simulink model "pack_96s"  (R2024b)
settings: Solver=ode4  StartTime=0.0  StopTime=T_stop  FixedStep=0.1  RelTol=1e-3
undefined symbols (not defined in the file): cell_dSoC_pct, cell_Q_Ah, cell_RO_scale, cp_coolant, h_rad, m_coolant, P_chiller_max, P_heater_max, T_cells_init, tau_chiller, tau_heater
settings Model: Creator=rayen  LastModifiedBy=rayen
settings OptimizationCC: ZeroExternalMemoryAtStartup=off  ZeroInternalMemoryAtStartup=off
settings DebuggingCC: AlgebraicLoopMsg=error
settings SFSimCC: SimTargetLang=C++
settings RTWCC: TargetLang=C++
settings GRTTargetCC: TargetLangStandard=C++11 (ISO)  CodeInterfacePackaging=C++ class

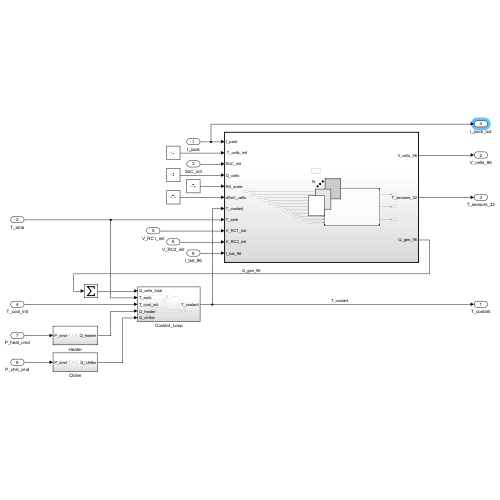
[thumbnail: Simulink's stored preview of the top-level diagram]
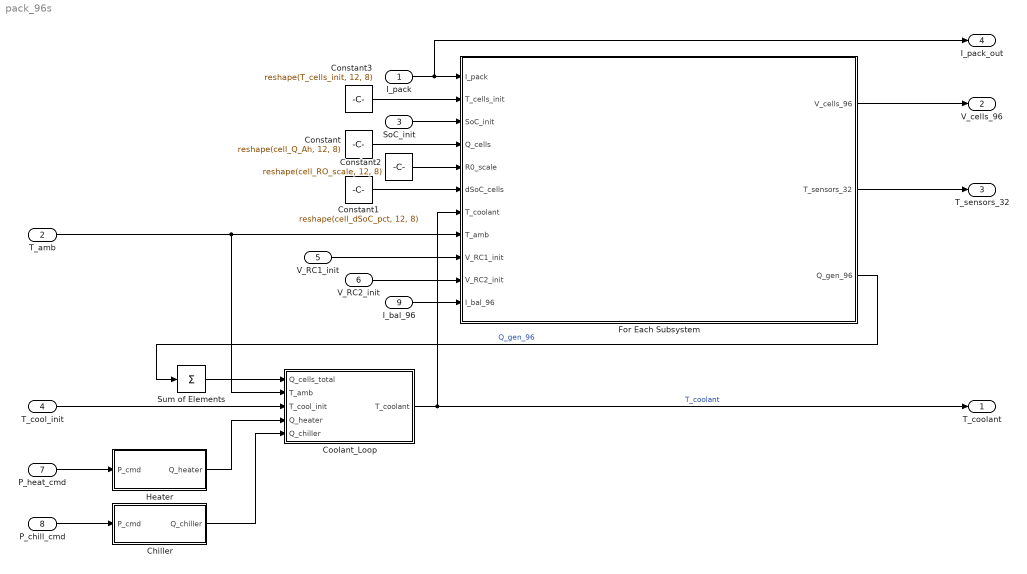
== system pack_96s ==
  I_pack : Inport  OutDataTypeStr=double
  T_amb : Inport  Port=2  OutDataTypeStr=double
  SoC_init : Inport  Port=3  OutDataTypeStr=double
  T_cool_init : Inport  Port=4  OutDataTypeStr=double
  V_RC1_init : Inport  Port=5  OutDataTypeStr=double
  V_RC2_init : Inport  Port=6  OutDataTypeStr=double
  P_heat_cmd : Inport  Port=7  OutDataTypeStr=double
  P_chill_cmd : Inport  Port=8  OutDataTypeStr=double
  I_bal_96 : Inport  Port=9  OutDataTypeStr=double
  Chiller : Subsystem
  Constant : Constant  Value=reshape(cell_Q_Ah, 12, 8)
  Constant1 : Constant  Value=reshape(cell_dSoC_pct, 12, 8)
  Constant2 : Constant  Value=reshape(cell_RO_scale, 12, 8)
  Constant3 : Constant  Value=reshape(T_cells_init, 12, 8)
  Coolant_Loop : Subsystem
  For Each Subsystem : Subsystem  TreatAsAtomicUnit=on
  Heater : Subsystem
  Sum of Elements : Sum  Inputs=+
  T_coolant : Outport  OutDataTypeStr=double
  V_cells_96 : Outport  Port=2  OutDataTypeStr=double
  T_sensors_32 : Outport  Port=3  OutDataTypeStr=double
  I_pack_out : Outport  Port=4  OutDataTypeStr=double
  wires:
  I_pack/1 -> I_pack_out/1, For Each Subsystem/1(I_pack)
  SoC_init/1 -> For Each Subsystem/3(SoC_init)
  Constant/1 -> For Each Subsystem/4(Q_cells)
  Constant2/1 -> For Each Subsystem/5(R0_scale)
  Constant1/1 -> For Each Subsystem/6(dSoC_cells)
  Sum of Elements/1 -> Coolant_Loop/1(Q_cells_total)
  Coolant_Loop/1(T_coolant) -> T_coolant/1, For Each Subsystem/7(T_coolant)  "T_coolant"
  Heater/1(Q_heater) -> Coolant_Loop/4(Q_heater)
  Chiller/1(Q_chiller) -> Coolant_Loop/5(Q_chiller)
  T_amb/1 -> For Each Subsystem/8(T_amb), Coolant_Loop/2(T_amb)
  T_cool_init/1 -> Coolant_Loop/3(T_cool_init)
  Constant3/1 -> For Each Subsystem/2(" T_cells_init")
  V_RC1_init/1 -> For Each Subsystem/9(V_RC1_init)
  V_RC2_init/1 -> For Each Subsystem/10(V_RC2_init)
  P_heat_cmd/1 -> Heater/1(P_cmd)
  P_chill_cmd/1 -> Chiller/1(P_cmd)
  For Each Subsystem/2(T_sensors_32) -> T_sensors_32/1
  For Each Subsystem/1(V_cells_96) -> V_cells_96/1
  For Each Subsystem/3(Q_gen_96) -> Sum of Elements/1  "Q_gen_96"
  I_bal_96/1 -> For Each Subsystem/11(I_bal_96)

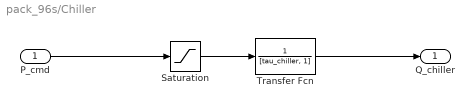
== system pack_96s/Chiller ==
  P_cmd : Inport
  Saturation : Saturate  UpperLimit=P_chiller_max  LowerLimit=0
  Transfer Fcn : TransferFcn  Denominator=[tau_chiller, 1]
  Q_chiller : Outport
  wires:
  Transfer Fcn/1 -> Q_chiller/1
  Saturation/1 -> Transfer Fcn/1
  P_cmd/1 -> Saturation/1

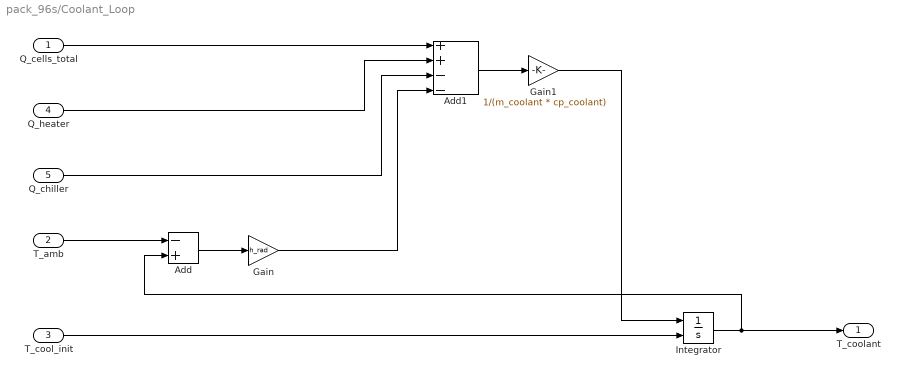
== system pack_96s/Coolant_Loop ==
  Q_cells_total : Inport
  T_amb : Inport  Port=2
  T_cool_init : Inport  Port=3
  Q_heater : Inport  Port=4
  Q_chiller : Inport  Port=5
  Add : Sum  Inputs=-+
  Add1 : Sum  Inputs=++--
  Gain : Gain  Gain=h_rad
  Gain1 : Gain  Gain=1/(m_coolant * cp_coolant)
  Integrator : Integrator  InitialConditionSource=external  LimitOutput=on  UpperSaturationLimit=80  LowerSaturationLimit=-40
  T_coolant : Outport
  wires:
  T_cool_init/1 -> Integrator/2
  Integrator/1 -> Add/2, T_coolant/1
  T_amb/1 -> Add/1
  Add/1 -> Gain/1
  Q_cells_total/1 -> Add1/1
  Q_heater/1 -> Add1/2
  Q_chiller/1 -> Add1/3
  Gain/1 -> Add1/4
  Add1/1 -> Gain1/1
  Gain1/1 -> Integrator/1

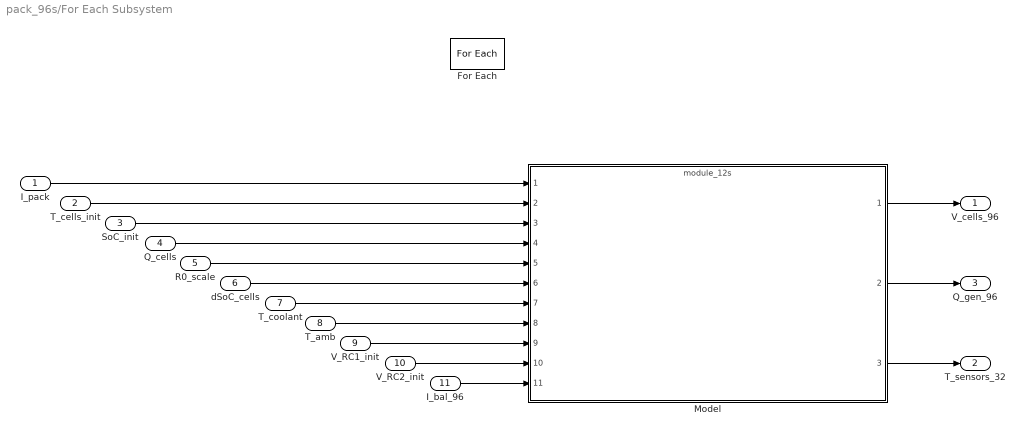
== system pack_96s/For Each Subsystem ==
  I_pack : Inport
  " T_cells_init" : Inport  Port=2  Partition=on  PartitionDimension=2  PartitionWidth=1  PartitionOffset=0
  SoC_init : Inport  Port=3
  Q_cells : Inport  Port=4  Partition=on  PartitionDimension=2  PartitionWidth=1  PartitionOffset=0
  R0_scale : Inport  Port=5  Partition=on  PartitionDimension=2  PartitionWidth=1  PartitionOffset=0
  dSoC_cells : Inport  Port=6  Partition=on  PartitionDimension=2  PartitionWidth=1  PartitionOffset=0
  T_coolant : Inport  Port=7
  T_amb : Inport  Port=8
  V_RC1_init : Inport  Port=9
  V_RC2_init : Inport  Port=10
  I_bal_96 : Inport  Port=11  Partition=on  PartitionDimension=2  PartitionWidth=1  PartitionOffset=0
  For Each : ForEach  DisableCoverage=on
  Model : ModelReference  ModelNameDialog=module_12s.slx  ModelReferenceVersion=1.48
  V_cells_96 : Outport  ConcatenationDimension=1
  T_sensors_32 : Outport  Port=2  ConcatenationDimension=1
  Q_gen_96 : Outport  Port=3  ConcatenationDimension=1
  wires:
  I_pack/1 -> Model/1
  Q_cells/1 -> Model/4
  SoC_init/1 -> Model/3
  " T_cells_init"/1 -> Model/2
  dSoC_cells/1 -> Model/6
  R0_scale/1 -> Model/5
  Model/3 -> T_sensors_32/1
  Model/1 -> V_cells_96/1
  T_coolant/1 -> Model/7
  T_amb/1 -> Model/8
  V_RC2_init/1 -> Model/10
  V_RC1_init/1 -> Model/9
  I_bal_96/1 -> Model/11
  Model/2 -> Q_gen_96/1

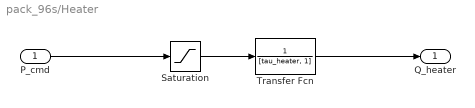
== system pack_96s/Heater ==
  P_cmd : Inport
  Saturation : Saturate  UpperLimit=P_heater_max  LowerLimit=0
  Transfer Fcn : TransferFcn  Denominator=[tau_heater, 1]
  Q_heater : Outport
  wires:
  P_cmd/1 -> Saturation/1
  Saturation/1 -> Transfer Fcn/1
  Transfer Fcn/1 -> Q_heater/1
